simulink model "quad_test_auto"  (R2018b)
settings: Solver=VariableStepAuto  StartTime=0.0  StopTime=20  RelTol=1e-3
undefined symbols (not defined in the file or in its folder): options
libraries: neural x348, simulink x3
(part 13 of 13)

== system quad_test_auto/nn_4/Layer 3/Delays 1 ==
  "p{3}" : Inport  PortDimensions=30
      mask Display: e = 0.06;c1 = [120 230 180]/255;c2 = ([120 230 180]+0)/(256+128);c3 = ([120 230 180]+128)/(256+128);patch([0 1 1 0],[0 0 1 1],c1);patch([0 1 1 1-e 1-e 0+e],[0 0 1 1-e 0+e 0+e],c2);patch([0 0 1 1-e 0+e 0+e],[0 1 1 1-e 1-e 0+e],c3);plot([0 1 1 0 0],[0 0 1 1 0]);
  mux : Mux  Inputs=1
      mask Display: e = 0.06;c1 = [120 150 230]/255;c2 = ([120 150 230]+0)/383;c3 = ([120 150 230]+128)/383;patch([0 1 1 0],[0 0 1 1],c1);patch([0 1 1 1-e 1-e 0+e],[0 0 1 1-e 0+e 0+e],c2);patch([0 0 1 1-e 0+e 0+e],[0 1 1 1-e 1-e 0+e],c3);plot([0 1 1 0 0],[0 0 1 1 0]);disp('Mux')
  "pd{3,2}" : Outport
      mask Display: e = 0.06;c1 = [120 230 180]/255;c2 = ([120 230 180]+0)/(256+128);c3 = ([120 230 180]+128)/(256+128);patch([0 1 1 0],[0 0 1 1],c1);patch([0 1 1 1-e 1-e 0+e],[0 0 1 1-e 0+e 0+e],c2);patch([0 0 1 1-e 0+e 0+e],[0 1 1 1-e 1-e 0+e],c3);plot([0 1 1 0 0],[0 0 1 1 0]);
  wires:
  "p{3}"/1 -> mux/1
  mux/1 -> "pd{3,2}"/1

== system quad_test_auto/nn_4/Layer 3/LW{3,2} ==
  "ad{3,2}" : Inport  PortDimensions=30
      mask Display: e = 0.06;c1 = [120 230 180]/255;c2 = ([120 230 180]+0)/(256+128);c3 = ([120 230 180]+128)/(256+128);patch([0 1 1 0],[0 0 1 1],c1);patch([0 1 1 1-e 1-e 0+e],[0 0 1 1-e 0+e 0+e],c2);patch([0 0 1 1-e 0+e 0+e],[0 1 1 1-e 1-e 0+e],c3);plot([0 1 1 0 0],[0 0 1 1 0]);
  "IW{3,2}(1,:)'" : Constant  Value=[0.431560290283934777644248015349148772656917572021484375;-0.33184494868527381061795722416718490421772003173828125;0.016764750860327949644190681510735885240137577056884765625;-0.371679745356561619384905270635499618947505950927734375;0.36131847970661901126021575691993348300457000732421875;-0.256967778600348639717054766151704825460910797119140625;-0.11513623902280743782622352000544196926057338714599609375;-0.46406121262294319773644701854209415614604949951171875;-0.25604817094496479246146236619097180664539337158203125;-0.08157315588575196618759122202391154132783412933349609375;0.3149443606509942927829115433269180357456207275390625;0.390670720909706725709753527553402818739414215087890625;0.362043363633431314330124450862058438360691070556640625;-0.276714433908025025932175822163117118179798126220703125;-0.04487808001421662862373551661221426911652088165283203125;-0.345068953814884504804894049811991862952709197998046875;0.390504030674442337289775650788214989006519317626953125;-0.05275649541217543314619575767210335470736026763916015625;-0.0034106678790755845000204349304340212256647646427154541015625;0.1841140406191839051786018899292685091495513916015625;-0.2275028275313683290281829840751015581190586090087890625;0.355384337674914896343381087717716582119464874267578125;0.1778948662073986664022839931931230239570140838623046875;-0.029359632210266682628141410305033787153661251068115234375;-0.1799629416635237511012945788024808280169963836669921875;-0.11697676369909505711408570505227544344961643218994140625;-0.1791646676574283336691451040678657591342926025390625;0.276594938384388033814076379712787456810474395751953125;0.378695734981777165639726945300935767590999603271484375;0.401469419577898334328125429237843491137027740478515625]
      mask Display: e = 0.06;c1 = [120 150 230]/255;c2 = ([120 150 230]+0)/383;c3 = ([120 150 230]+128)/383;patch([0 1 1 0],[0 0 1 1],c1);patch([0 1 1 1-e 1-e 0+e],[0 0 1 1-e 0+e 0+e],c2);patch([0 0 1 1-e 0+e 0+e],[0 1 1 1-e 1-e 0+e],c3);plot([0 1 1 0 0],[0 0 1 1 0]);disp('weights');
  Mux : Mux  Inputs=1
      mask Display: e = 0.06;c1 = [120 150 230]/255;c2 = ([120 150 230]+0)/383;c3 = ([120 150 230]+128)/383;patch([0 1 1 0],[0 0 1 1],c1);patch([0 1 1 1-e 1-e 0+e],[0 0 1 1-e 0+e 0+e],c2);patch([0 0 1 1-e 0+e 0+e],[0 1 1 1-e 1-e 0+e],c3);plot([0 1 1 0 0],[0 0 1 1 0]);disp('Mux');
  dotprod1 : neural/Weight Functions/dotprod
  "lz{3,2}" : Outport
      mask Display: e = 0.06;c1 = [120 230 180]/255;c2 = ([120 230 180]+0)/(256+128);c3 = ([120 230 180]+128)/(256+128);patch([0 1 1 0],[0 0 1 1],c1);patch([0 1 1 1-e 1-e 0+e],[0 0 1 1-e 0+e 0+e],c2);patch([0 0 1 1-e 0+e 0+e],[0 1 1 1-e 1-e 0+e],c3);plot([0 1 1 0 0],[0 0 1 1 0]);
  wires:
  "IW{3,2}(1,:)'"/1 -> dotprod1/1
  "ad{3,2}"/1 -> dotprod1/2
  dotprod1/1 -> Mux/1
  Mux/1 -> "lz{3,2}"/1

== matlab function quad_test_auto/MATLAB Function ==
  data: r1 input; F output; r2 input; r3 input; x3 input; x6 input; x7 input; x8 input; x10 input; x11 input; tau_phi output; tau_theta output; tau_psi output
function [F,tau_phi,tau_theta,tau_psi] = fcn(r1,r2,r3,x3,x6,x7,x8,x10,x11)
%initialization
m=1.4;
g=9.81;
F= m*g-10*(x3-r1)+3*x6;
tau_phi=-(x7-r2)-x10;
tau_theta=-(x8-r3)-x11;
tau_psi=0;
